simulink model "fmi_setup_test_1"  (R2021b)
settings: Solver=FixedStepAuto  StartTime=0.0  StopTime=10.0  RelTol=1e-3  EnableMultiTasking=on
PreLoadFcn:
  | fmi_setup_init
libraries: spspowerguiLib x1
settings Model: Creator=lordx  LastModifiedBy=lordx
settings DataIOCC: SaveFormat=Array
settings OptimizationCC: UseDivisionForNetSlopeComputation=on  DefaultUnderspecifiedDataType=single  EnhancedBackFolding=on  EnableMemcpy=off  PassReuseOutputArgsThreshold=0  OptimizeBlockOrder=speed  DifferentSizesBufferReuse=on
settings DebuggingCC: ParameterTunabilityLossMsg=error  DebugExecutionForFMUViaOutOfProcess=on
settings HardwareCC: ProdBitPerPointer=32  ProdBitPerSizeT=32  ProdBitPerPtrDiffT=32  ProdWordSize=32  ProdHWDeviceType=Intel->x86-32 (Windows32)  TargetBitPerPointer=64  TargetBitPerSizeT=64  TargetBitPerPtrDiffT=64  TargetLongLongMode=on  TargetIntDivRoundTo=Zero  TargetEndianess=LittleEndian  TargetWordSize=64  TargetHWDeviceType=MATLAB Host  ProdEqTarget=off
settings ModelReferenceCC: EnableRefExpFcnMdlSchedulingChecks=off  PropagateVarSize=During execution  PropagateSignalLabelsOutOfModel=off
settings SFSimCC: MATLABDynamicMemAlloc=off
settings RTWCC: Description=FMU based on GRT (Functional Mock-up Unit)  SystemTargetFile=grtfmi.tlc  GenerateMakefile=off  TemplateMakefile=none  GenerateReport=on  RetainRTWFile=on  LaunchReport=on
settings CodeAppCC: ForceParamTrailComments=on  OperatorAnnotations=on  StateflowObjectComments=on  MATLABSourceComments=on
settings STFCustomTargetCC: TargetLangStandard=C99 (ISO)  CombineOutputUpdateFcns=on  GRTInterface=off  SystemTargetFile=grtfmi.tlc
settings GRTTargetCC: ParMdlRefBuildCompliant=off  CompOptLevelCompliant=off  ConcurrentExecutionCompliant=off  MatFileLogging=off  CPPClassGenCompliant=off  UseToolchainInfoCompliant=off  RTWCAPISignals=on  RTWCAPIParams=on  RTWCAPIStates=on  RTWCAPIRootIO=on

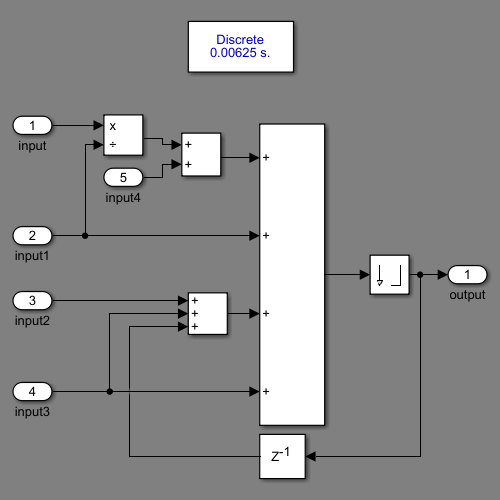
[thumbnail: Simulink's stored preview of the top-level diagram]
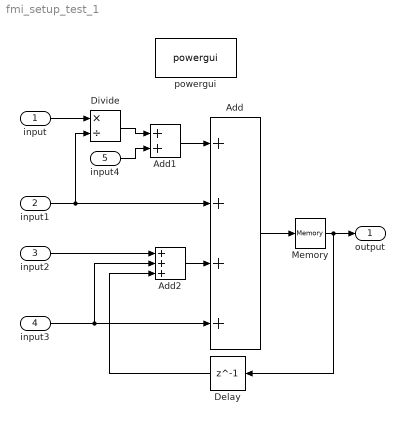
== system fmi_setup_test_1 ==
  input : Inport
  input1 : Inport  Port=2
  input2 : Inport  Port=3
  input3 : Inport  Port=4
  input4 : Inport  Port=5
  Add : Sum  Inputs=++++
  Add1 : Sum
  Add2 : Sum  Inputs=+++
  Delay : Delay  DelayLength=1
  Divide : Product  Inputs=*/
  Memory : Memory
  powergui : spspowerguiLib/powergui  Priority=1  SimulationMode=Discrete  SampleTime=6.25e-3  frequency=60  Iterations=50  frequencyindice=60  Pbase=100e6  ErrMax=1e-4  UnitsV=kV  UnitsW=MW  buscounter=0  FunctionMessages=off  echomessages=off  EnableUseOfTLC=off  CurrentSourceSwitches=off  DisableSnubberDevices=off  DisableRonSwitches=off  DisableVfSwitches=off  DisplayEquations=off  AutomaticDiscreteSolvers=off  SolverType=Tustin/Backward Euler (TBE)  Interpol=off  ExternalGateDelay=off  methode=off  Ts=100  x0status=blocks  SPID=on  SwTol=0  HookPort=off  NonlinearTolerance=1e-4  nMaxIteration=100  ContinueOnMaxIteration=off  RestoreLinks=warning  ResistiveCurrentMeasurement=off  Frange=[0:2:500]  Ylog=off  Xlog=on  ShowGrid=off  save=off  variable=ZData  structure=0  ZoomFFT=off  StartTime=0.0  cycles=1  DisplayStyle=1  fundamental=60  FreqAxis=off  MaxFrequency=1000  frequencyindicesteady=1  RmsSteady=1  display=off
  output : Outport
  wires:
  input/1 -> Divide/1
  input1/1 -> Divide/2, Add/2
  Add/1 -> Memory/1
  input2/1 -> Add2/1
  Add2/1 -> Add/3
  Divide/1 -> Add1/1
  input4/1 -> Add1/2
  Add1/1 -> Add/1
  input3/1 -> Add2/2, Add/4
  Memory/1 -> Delay/1, output/1
  Delay/1 -> Add2/3
